simulink library "dcpctrl"  (R2016b)
settings: Solver=ode45  StartTime=0.0  StopTime=10.0  RelTol=1e-3  EnableMultiTasking=on
undefined symbols (not defined in the file): Humusoft, MF644, robot, ts
libraries: simulink x42, sldrtlib x11, dspsigops x2
settings Model: Creator=julianleland  LastModifiedBy=julianleland
settings DataIOCC: LimitDataPoints=on
settings OptimizationCC: LifeSpan=inf
settings DebuggingCC: AllowSymbolicDim=off  SFUnexpectedBacktrackingDiag=warning  SFNoUnconditionalDefaultTransitionDiag=warning  SFExecutionAtInitializationDiag=none
settings GRTTargetCC: TargetLangStandard=C89/C90 (ANSI)  GeneratePreprocessorConditionals=Disable all
settings ConfigComp: CovMetricSettings=dw  CovHtmlReporting=on  CovSaveCumulativeToWorkspaceVar=on  CovSaveSingleToWorkspaceVar=on  CovExternalEMLEnable=off

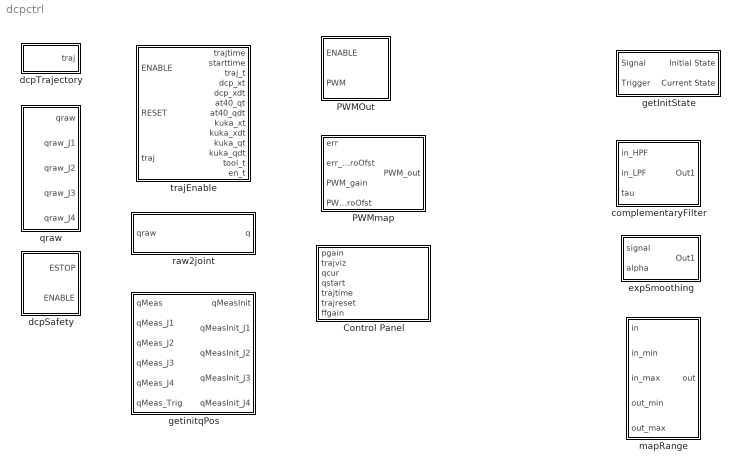
== system dcpctrl ==
  Control Panel : Subsystem
  PWMOut : Subsystem
  PWMmap : Subsystem  mask(PWMmap){}
      mask help:
      | Translates an error signal into a PWM signal, accounting for the dynamics of the AT40GW's PWM interface (deadband, saturation errors).
      |
      | Inputs:
      |  - err: Error signal, unscaled. 4 channels wide.
      |  - err_zeroOfst: Adjusts error "zero" band. A positive number X at this port will cause error values within X of zero to be treated as zero. Default input should be zero.
      |  - PWM_gain: Gain term applied to error signal before conversion to PWM signal. Use this input to scale all PWM signals. Default input should be 1
      |  - PWM_zeroOfst: Adjusts offset of deadband. Positive values will cause deadband limits to increase or decrease. Default input should be zero.
  complementaryFilter : Subsystem
  dcpSafety : Subsystem
  dcpTrajectory : Subsystem
  expSmoothing : Subsystem
  getInitState : Subsystem
  getinitqPos : Subsystem
  "mapRange " : MATLAB Function  TreatAsAtomicUnit=on
  qraw : Subsystem
  raw2joint : Subsystem
  trajEnable : Subsystem

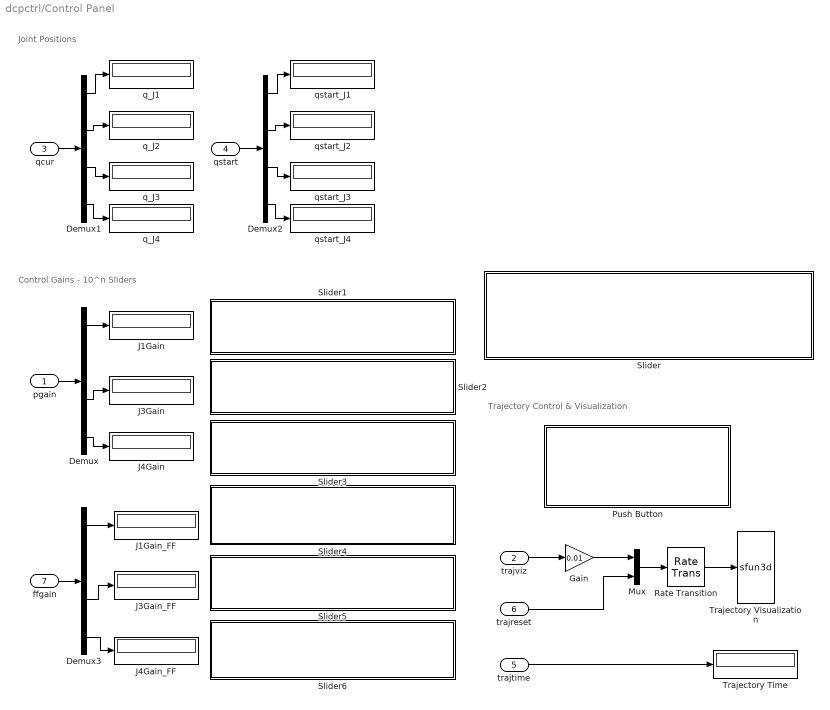
== system dcpctrl/Control Panel ==
  note: Control Gains - 10^n Sliders
  note: Trajectory Control & Visualization
  note: Joint Positions
  pgain : Inport
  trajviz : Inport  Port=2
  qcur : Inport  Port=3
  qstart : Inport  Port=4
  trajtime : Inport  Port=5
  trajreset : Inport  Port=6
  ffgain : Inport  Port=7
  Demux{,1..3} (4 alike) : Demux
  Gain : Gain  Gain=0.01
  J1Gain : Display
  J1Gain_FF : Display
  J3Gain : Display
  J3Gain_FF : Display
  J4Gain : Display
  J4Gain_FF : Display
  Mux : Mux  Inputs=2
  Push Button : Subsystem  DialogController=hmiCreateDDGDialog  IsWebBlock=on  mask(MWDashboardBlock){webBlockId=d14440dc-dcfb-4a22-9820-9883405fda4f, webBlockType=pushbutton, ShowInLibBrwoser=on, ShowInitialText=on, HMISrcModelName=[]}
      mask prompts: webBlockId "WebBlock Id"; webBlockType "WebBlock Type"; HMISrcModelName "Source Model"
      mask Help: helpview([docroot '/mapfiles/simulink.map'], 'hmi_push_button')
      mask Display:
      | model = bdroot(gcb);
      | if strcmp(get_param(model,'BlockDiagramType'), 'library')
      |     image([(matlabroot) '/toolbox/simulink/hmi/icons/PushButton.png']);
      | end
  Rate Transition : RateTransition
  Slider : Subsystem  DialogController=hmiCreateDDGDialog  IsWebBlock=on  mask(MWDashboardBlock){webBlockId=f0c68e46-865a-4d96-89a7-5e1e8ebc446d, webBlockType=slider, ShowInLibBrowser=on, ShowInitialText=on, HMISrcModelName=[]}
      mask prompts: webBlockId "WebBlock Id"; webBlockType "WebBlock Type"; HMISrcModelName "Source Model"
      mask Help: helpview([docroot '/mapfiles/simulink.map'], 'hmi_slider')
      mask Display:
      | if strcmp(get_param(bdroot(gcb),'BlockDiagramType'), 'library')
      |     image([(matlabroot) '/toolbox/simulink/hmi/icons/Slider.png']);
      | end
  Slider1 : Subsystem  DialogController=hmiCreateDDGDialog  IsWebBlock=on  mask(MWDashboardBlock){webBlockId=1b4d9833-0382-4353-be8c-f20f38eb9aab, webBlockType=slider, ShowInLibBrowser=on, ShowInitialText=on, HMISrcModelName=[]}
      mask prompts: webBlockId "WebBlock Id"; webBlockType "WebBlock Type"; HMISrcModelName "Source Model"
      mask Help: helpview([docroot '/mapfiles/simulink.map'], 'hmi_slider')
      mask Display:
      | if strcmp(get_param(bdroot(gcb),'BlockDiagramType'), 'library')
      |     image([(matlabroot) '/toolbox/simulink/hmi/icons/Slider.png']);
      | end
  Slider2 : Subsystem  DialogController=hmiCreateDDGDialog  IsWebBlock=on  mask(MWDashboardBlock){webBlockId=cbf9babb-b489-42eb-b20a-0d2a912eb983, webBlockType=slider, ShowInLibBrowser=on, ShowInitialText=on, HMISrcModelName=[]}
      mask prompts: webBlockId "WebBlock Id"; webBlockType "WebBlock Type"; HMISrcModelName "Source Model"
      mask Help: helpview([docroot '/mapfiles/simulink.map'], 'hmi_slider')
      mask Display:
      | if strcmp(get_param(bdroot(gcb),'BlockDiagramType'), 'library')
      |     image([(matlabroot) '/toolbox/simulink/hmi/icons/Slider.png']);
      | end
  Slider3 : Subsystem  DialogController=hmiCreateDDGDialog  IsWebBlock=on  mask(MWDashboardBlock){webBlockId=af3345d3-46b3-4b00-a2f8-3f6dd7fd4884, webBlockType=slider, ShowInLibBrowser=on, ShowInitialText=on, HMISrcModelName=[]}
      mask prompts: webBlockId "WebBlock Id"; webBlockType "WebBlock Type"; HMISrcModelName "Source Model"
      mask Help: helpview([docroot '/mapfiles/simulink.map'], 'hmi_slider')
      mask Display:
      | if strcmp(get_param(bdroot(gcb),'BlockDiagramType'), 'library')
      |     image([(matlabroot) '/toolbox/simulink/hmi/icons/Slider.png']);
      | end
  Slider4 : Subsystem  DialogController=hmiCreateDDGDialog  IsWebBlock=on  mask(MWDashboardBlock){webBlockId=c89750c1-d32c-4c6a-899a-daca88898995, webBlockType=slider, ShowInLibBrowser=on, ShowInitialText=on, HMISrcModelName=[]}
      mask prompts: webBlockId "WebBlock Id"; webBlockType "WebBlock Type"; HMISrcModelName "Source Model"
      mask Help: helpview([docroot '/mapfiles/simulink.map'], 'hmi_slider')
      mask Display:
      | if strcmp(get_param(bdroot(gcb),'BlockDiagramType'), 'library')
      |     image([(matlabroot) '/toolbox/simulink/hmi/icons/Slider.png']);
      | end
  Slider5 : Subsystem  DialogController=hmiCreateDDGDialog  IsWebBlock=on  mask(MWDashboardBlock){webBlockId=a8dd70f1-7c39-409c-bbaa-299b93baa409, webBlockType=slider, ShowInLibBrowser=on, ShowInitialText=on, HMISrcModelName=[]}
      mask prompts: webBlockId "WebBlock Id"; webBlockType "WebBlock Type"; HMISrcModelName "Source Model"
      mask Help: helpview([docroot '/mapfiles/simulink.map'], 'hmi_slider')
      mask Display:
      | if strcmp(get_param(bdroot(gcb),'BlockDiagramType'), 'library')
      |     image([(matlabroot) '/toolbox/simulink/hmi/icons/Slider.png']);
      | end
  Slider6 : Subsystem  DialogController=hmiCreateDDGDialog  IsWebBlock=on  mask(MWDashboardBlock){webBlockId=99b5f6f1-a2e8-44e0-a565-9b4153c34515, webBlockType=slider, ShowInLibBrowser=on, ShowInitialText=on, HMISrcModelName=[]}
      mask prompts: webBlockId "WebBlock Id"; webBlockType "WebBlock Type"; HMISrcModelName "Source Model"
      mask Help: helpview([docroot '/mapfiles/simulink.map'], 'hmi_slider')
      mask Display:
      | if strcmp(get_param(bdroot(gcb),'BlockDiagramType'), 'library')
      |     image([(matlabroot) '/toolbox/simulink/hmi/icons/Slider.png']);
      | end
  Trajectory Time : Display
  Trajectory Visualization : S-Function  LoadFcn=if exist('sfun3d','file'), sfun3d([],[],[],'LoadBlock'); end  FunctionName=sfun3d  Parameters=ax,T,np,cp,gd,ls,mk  SFunctionDeploymentMode=off  EnableBusSupport=off  mask(3D Graph){np=2, ax=[30 80 -20 20 -10 30], cp=[80 10 20], gd=on, ls=-, mk=., T=0.1}
      mask prompts: np "Number of point (lines)"; ax "[xmin xmax  ymin ymax zmin zmax]"; cp "Camera position (use [0 0 1] for 2D XY view)"; gd "Grid (on|off)"; ls "LineStyle"; mk "Marker"; T "Sampling Time"
      mask help:
      | This block plots the position of several points in the XYZ space. The input contains the coordinates of all the points (x1,y1,z1,x2,y2,z2,...).
      | The number of points (lines), the XYZ ranges, camera position, grid, linestyle, marker and sampling time, can be set as mask parameters.
      settings: CopyFcn=if exist('sfun3d','file'), sfun3d([],[],[],'CopyBlock'); end  DeleteFcn=if exist('sfun3d','file'), sfun3d([],[],[],'DeleteBlock'); end  NameChangeFcn=if exist('sfun3d','file'), sfun3d([],[],[],'NameChange'); end
      mask Help:
      | This block plots the position of several points in the XYZ space. The input contains the coordinates of all the points (x1,y1,z1,x2,y2,z2,...).
      | The number of points (lines), the XYZ ranges, camera position, grid, linestyle, marker and sampling time, can be set as mask parameters.
      mask TypeOptions ls: - | -- | : | -. | none
      mask TypeOptions mk: none | . | + | o | * | x | square | diamond | v | ^ | > | < | pentagram | hexagram
      mask Display: plot([.05 .95 .95 .05 .05],[.45 .45 .95 .95 .45], 0.5+cos(0:0.1:2*pi)*0.3,0.7+sin(0:0.1:2*pi)*0.2)
  q_J{1..4} (4 alike) : Display
  qstart_J{1..4} (4 alike) : Display
  wires:
  trajreset/1 -> Mux/2
  Rate Transition/1 -> Trajectory Visualization/1
  Mux/1 -> Rate Transition/1
  Gain/1 -> Mux/1
  trajviz/1 -> Gain/1
  Demux3/3 -> J3Gain_FF/1
  Demux3/1 -> J1Gain_FF/1
  Demux3/4 -> J4Gain_FF/1
  ffgain/1 -> Demux3/1
  trajtime/1 -> Trajectory Time/1
  Demux2/2 -> qstart_J2/1
  Demux2/3 -> qstart_J3/1
  Demux2/1 -> qstart_J1/1
  Demux2/4 -> qstart_J4/1
  qstart/1 -> Demux2/1
  Demux1/2 -> q_J2/1
  Demux1/3 -> q_J3/1
  Demux1/1 -> q_J1/1
  Demux1/4 -> q_J4/1
  qcur/1 -> Demux1/1
  Demux/3 -> J3Gain/1
  Demux/1 -> J1Gain/1
  Demux/4 -> J4Gain/1
  pgain/1 -> Demux/1

== system dcpctrl/PWMOut ==
  ENABLE : Inport
  "PWM " : Inport  Port=2
  Demux : Demux
  PWM_zero : Constant  Value=robot.Joint(:).PWM_zero
  Switch : Switch  Criteria=u2 ~= 0
  T0Out_PWM : sldrtlib/Frequency Output  SampleTime=-1  MaxMissedTicks=10  ShowMissedTicks=off  YieldWhenWaiting=off  DrvName=Humusoft/MF644  DrvAddress=4294967295  DrvOptions=585  Channels=1  FrequencySource=1  Frequency=500  FrequencyFinalValue=[]  DutySource=2  Duty=0.5  DutyFinalValue=0.5
      settings: AttributesFormatString=Humusoft\nMF644 [auto]
  T1Out_PWM : sldrtlib/Frequency Output  SampleTime=-1  MaxMissedTicks=10  ShowMissedTicks=off  YieldWhenWaiting=off  DrvName=Humusoft/MF644  DrvAddress=4294967295  DrvOptions=585  Channels=2  FrequencySource=1  Frequency=500  FrequencyFinalValue=[]  DutySource=2  Duty=0.5  DutyFinalValue=0.5
      settings: AttributesFormatString=Humusoft\nMF644 [auto]
  T2Out_PWM : sldrtlib/Frequency Output  SampleTime=-1  MaxMissedTicks=10  ShowMissedTicks=off  YieldWhenWaiting=off  DrvName=Humusoft/MF644  DrvAddress=4294967295  DrvOptions=585  Channels=3  FrequencySource=1  Frequency=500  FrequencyFinalValue=[]  DutySource=2  Duty=0.5  DutyFinalValue=0.5
      settings: AttributesFormatString=Humusoft\nMF644 [auto]
  T3Out_PWM : sldrtlib/Frequency Output  SampleTime=-1  MaxMissedTicks=10  ShowMissedTicks=off  YieldWhenWaiting=off  DrvName=Humusoft/MF644  DrvAddress=4294967295  DrvOptions=585  Channels=4  FrequencySource=1  Frequency=500  FrequencyFinalValue=[]  DutySource=2  Duty=0.5  DutyFinalValue=0.5
      settings: AttributesFormatString=Humusoft\nMF644 [auto]
  wires:
  ENABLE/1 -> Switch/2
  PWM_zero/1 -> Switch/3
  "PWM "/1 -> Switch/1
  Switch/1 -> Demux/1
  Demux/1 -> T0Out_PWM/1
  Demux/2 -> T1Out_PWM/1
  Demux/3 -> T2Out_PWM/1
  Demux/4 -> T3Out_PWM/1

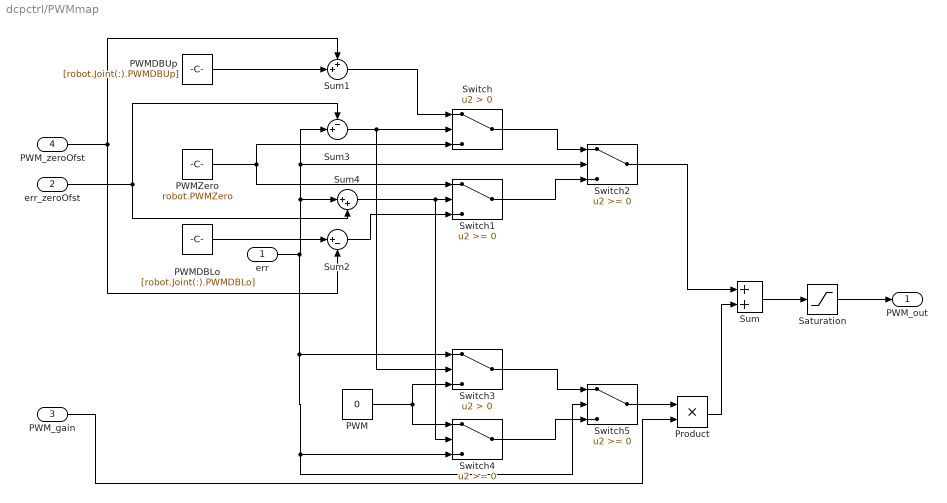
== system dcpctrl/PWMmap ==
  err : Inport
  err_zeroOfst : Inport  Port=2
  "PWM_gain " : Inport  Port=3
  PWM_zeroOfst : Inport  Port=4
  PWM : Constant  Value=0
  PWMDBLo : Constant  Value=[robot.Joint(:).PWMDBLo]
  PWMDBUp : Constant  Value=[robot.Joint(:).PWMDBUp]
  PWMZero : Constant  Value=robot.PWMZero
  Product : Product
  Saturation : Saturate  UpperLimit=[robot.Joint(:).PWMDBMax]  LowerLimit=[robot.Joint(:).PWMDBMin]
  Sum : Sum
  Sum1 : Sum  Inputs=++|
  Sum2 : Sum  Inputs=|+-
  Sum3 : Sum  Inputs=-+|
  Sum4 : Sum  Inputs=|++
  Switch : Switch  Criteria=u2 > Threshold
  Switch{1..2,4..5} (4 alike) : Switch
  Switch3 : Switch  Criteria=u2 > Threshold
  PWM_out : Outport
  wires:
  Switch2/1 -> Sum/1
  Product/1 -> Sum/2
  Sum/1 -> Saturation/1
  Switch5/1 -> Product/1
  PWM/1 -> Switch3/3, Switch4/1
  Switch4/1 -> Switch5/3
  Switch3/1 -> Switch5/1
  Sum1/1 -> Switch/1
  Switch1/1 -> Switch2/3
  Switch/1 -> Switch2/1
  Sum3/1 -> Switch/2, Switch3/2
  Sum4/1 -> Switch1/2, Switch4/2
  err_zeroOfst/1 -> Sum3/1, Sum4/2
  Sum2/1 -> Switch1/3
  PWMDBLo/1 -> Sum2/1
  PWMDBUp/1 -> Sum1/2
  err/1 -> Sum3/2, Switch2/2, Sum4/1, Switch5/2, Switch4/3, Switch3/1
  PWM_zeroOfst/1 -> Sum2/2, Sum1/1
  PWMZero/1 -> Switch/3, Switch1/1
  Saturation/1 -> PWM_out/1
  "PWM_gain "/1 -> Product/2

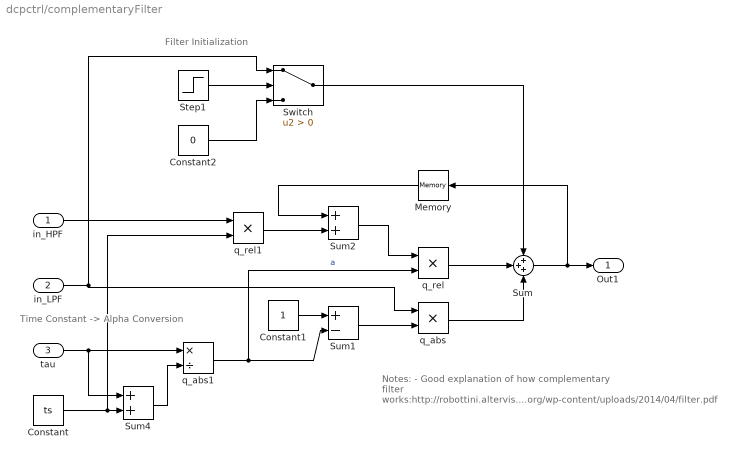
== system dcpctrl/complementaryFilter ==
  note: Notes:
      | - Good explanation of how complementary filter works:http://robottini.altervista.org/wp-content/uploads/2014/04/filter.pdf
  note: Filter Initialization
  note: Time Constant -> Alpha Conversion
  in_HPF : Inport
  "in_LPF " : Inport  Port=2
  tau : Inport  Port=3
  Constant : Constant  Value=ts
  Constant1 : Constant
  Constant2 : Constant  Value=0
  Memory : Memory
  Step1 : Step  Time=ts  Before=1  After=0  SampleTime=0
  Sum : Sum  Inputs=+++
  Sum1 : Sum  Inputs=+-
  Sum2 : Sum
  Sum4 : Sum
  Switch : Switch  Criteria=u2 > Threshold
  q_abs : Product
  q_abs1 : Product  Inputs=*/
  q_rel : Product
  q_rel1 : Product
  Out1 : Outport
  wires:
  Step1/1 -> Switch/2
  Constant2/1 -> Switch/3
  Switch/1 -> Sum/1
  in_HPF/1 -> q_rel1/1
  q_rel1/1 -> Sum2/2
  Constant/1 -> Sum4/2, q_rel1/2
  q_abs1/1 -> Sum1/2, q_rel/2  "a"
  Sum4/1 -> q_abs1/2
  tau/1 -> Sum4/1, q_abs1/1
  Memory/1 -> Sum2/1
  Sum2/1 -> q_rel/1
  q_rel/1 -> Sum/2
  q_abs/1 -> Sum/3
  Constant1/1 -> Sum1/1
  "in_LPF "/1 -> Switch/1, q_abs/1
  Sum1/1 -> q_abs/2
  Sum/1 -> Out1/1, Memory/1

== system dcpctrl/dcpSafety ==
  DIO_ESTOP : sldrtlib/Digital Input  SampleTime=-1  MaxMissedTicks=10  ShowMissedTicks=off  YieldWhenWaiting=off  DrvName=Humusoft/MF644  DrvAddress=4294967295  DrvOptions=585  Channels=1  BitMode=1  DataType=9
      settings: AttributesFormatString=Humusoft\nMF644 [auto]
  DIO_Enable : sldrtlib/Digital Input  SampleTime=-1  MaxMissedTicks=10  ShowMissedTicks=off  YieldWhenWaiting=off  DrvName=Humusoft/MF644  DrvAddress=4294967295  DrvOptions=585  Channels=2  BitMode=1  DataType=9
      settings: AttributesFormatString=Humusoft\nMF644 [auto]
  Logical Operator : Logic  Operator=NOT  AllPortsSameDT=off  OutDataTypeStr=boolean
  ESTOP : Outport
  ENABLE : Outport  Port=2
  wires:
  DIO_ESTOP/1 -> ESTOP/1
  DIO_Enable/1 -> Logical Operator/1
  Logical Operator/1 -> ENABLE/1

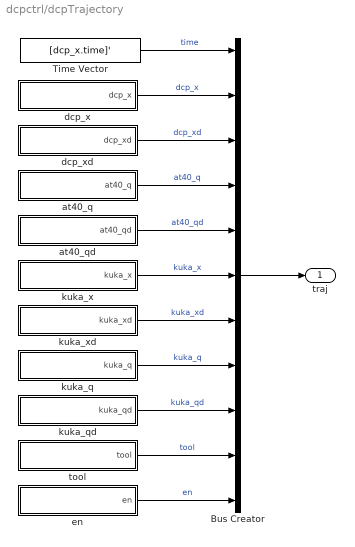
== system dcpctrl/dcpTrajectory ==
  Bus Creator : BusCreator  Inputs=11
  Time Vector : FromWorkspace  VariableName=[dcp_x.time]'  SampleTime=0
  at40_q : Subsystem
  at40_qd : Subsystem
  dcp_x : Subsystem
  dcp_xd : Subsystem
  en : Subsystem
  kuka_q : Subsystem
  kuka_qd : Subsystem
  kuka_x : Subsystem
  kuka_xd : Subsystem
  tool : Subsystem
  traj : Outport
  wires:
  dcp_x/1(dcp_x) -> Bus Creator/2  "dcp_x"
  en/1(en) -> Bus Creator/11  "en"
  tool/1(tool) -> Bus Creator/10  "tool"
  kuka_qd/1(kuka_qd) -> Bus Creator/9  "kuka_qd"
  kuka_q/1(kuka_q) -> Bus Creator/8  "kuka_q"
  kuka_xd/1(kuka_xd) -> Bus Creator/7  "kuka_xd"
  kuka_x/1(kuka_x) -> Bus Creator/6  "kuka_x"
  at40_q/1(at40_q) -> Bus Creator/4  "at40_q"
  Time Vector/1 -> Bus Creator/1  "time"
  dcp_xd/1(dcp_xd) -> Bus Creator/3  "dcp_xd"
  at40_qd/1(at40_qd) -> Bus Creator/5  "at40_qd"
  Bus Creator/1 -> traj/1

== system dcpctrl/expSmoothing ==
  signal : Inport
  alpha : Inport  Port=2
  Constant : Constant
  Memory : Memory
  Product : Product
  Product1 : Product
  Subtract : Sum  Inputs=+-
  Sum : Sum  Inputs=|++
  Out1 : Outport
  wires:
  Subtract/1 -> Product/2
  signal/1 -> Product1/1
  Memory/1 -> Product/1
  alpha/1 -> Subtract/2, Product1/2
  Product1/1 -> Sum/1
  Product/1 -> Sum/2
  Sum/1 -> Out1/1, Memory/1
  Constant/1 -> Subtract/1

== system dcpctrl/getInitState ==
  Signal : Inport
  Trigger : Inport  Port=2
  Delay : Delay  DelayLength=1  InitialCondition=0
  Enabled Subsystem : Subsystem  TreatAsAtomicUnit=on
  Initial State : Outport
  Current State : Outport  Port=2
  wires:
  Delay/1 -> Enabled Subsystem/1(Trigger)
  Trigger/1 -> Enabled Subsystem/Enable, Delay/1
  Enabled Subsystem/2(Cur_State) -> Current State/1
  Enabled Subsystem/1(Init_State) -> Initial State/1
  Signal/1 -> Enabled Subsystem/2(Signal)

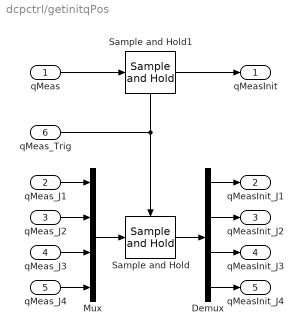
== system dcpctrl/getinitqPos ==
  qMeas : Inport
  qMeas_J1 : Inport  Port=2
  qMeas_J2 : Inport  Port=3
  qMeas_J3 : Inport  Port=4
  qMeas_J4 : Inport  Port=5
  qMeas_Trig : Inport  Port=6
  Demux : Demux
  Mux : Mux
  Sample and Hold : dspsigops/Sample and Hold  trig=Rising edge  initCond=0  latchinput=off
  Sample and Hold1 : dspsigops/Sample and Hold  trig=Rising edge  initCond=0  latchinput=off
  qMeasInit : Outport
  qMeasInit_J1 : Outport  Port=2
  qMeasInit_J2 : Outport  Port=3
  qMeasInit_J3 : Outport  Port=4
  qMeasInit_J4 : Outport  Port=5
  wires:
  qMeas_Trig/1 -> Sample and Hold/Trigger, Sample and Hold1/Trigger
  qMeas_J4/1 -> Mux/4
  qMeas_J3/1 -> Mux/3
  qMeas_J2/1 -> Mux/2
  qMeas_J1/1 -> Mux/1
  Demux/2 -> qMeasInit_J2/1
  Demux/3 -> qMeasInit_J3/1
  Demux/4 -> qMeasInit_J4/1
  Demux/1 -> qMeasInit_J1/1
  Sample and Hold/1 -> Demux/1
  Mux/1 -> Sample and Hold/1
  Sample and Hold1/1 -> qMeasInit/1
  qMeas/1 -> Sample and Hold1/1

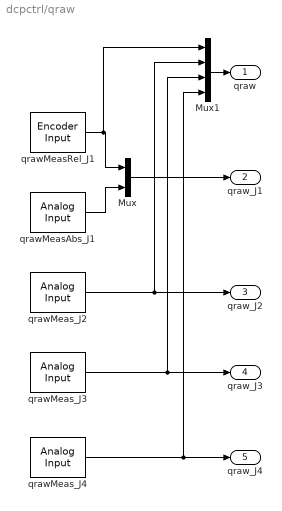
== system dcpctrl/qraw ==
  Mux : Mux  Inputs=2
  Mux1 : Mux
  qrawMeasAbs_J1 : sldrtlib/Analog Input  SampleTime=-1  MaxMissedTicks=10  ShowMissedTicks=off  YieldWhenWaiting=off  DrvName=Humusoft/MF644  DrvAddress=4294967295  DrvOptions=585  Channels=1  RangeMode=1  VoltRange=1  DataType=1
      settings: AttributesFormatString=Humusoft\nMF644 [auto]
  qrawMeasRel_J1 : sldrtlib/Encoder Input  SampleTime=-1  MaxMissedTicks=10  ShowMissedTicks=off  YieldWhenWaiting=off  DrvName=Humusoft/MF644  DrvAddress=4294967295  DrvOptions=585  Channels=1  QuadMode=3  IndexPulse=2  InputFilter=Inf  DataType=1
      settings: AttributesFormatString=Humusoft\nMF644 [auto]
  qrawMeas_J2 : sldrtlib/Analog Input  SampleTime=-1  MaxMissedTicks=10  ShowMissedTicks=off  YieldWhenWaiting=off  DrvName=Humusoft/MF644  DrvAddress=4294967295  DrvOptions=585  Channels=2  RangeMode=1  VoltRange=1  DataType=1
      settings: AttributesFormatString=Humusoft\nMF644 [auto]
  qrawMeas_J3 : sldrtlib/Analog Input  SampleTime=-1  MaxMissedTicks=10  ShowMissedTicks=off  YieldWhenWaiting=off  DrvName=Humusoft/MF644  DrvAddress=4294967295  DrvOptions=585  Channels=3  RangeMode=1  VoltRange=1  DataType=1
      settings: AttributesFormatString=Humusoft\nMF644 [auto]
  qrawMeas_J4 : sldrtlib/Analog Input  SampleTime=-1  MaxMissedTicks=10  ShowMissedTicks=off  YieldWhenWaiting=off  DrvName=Humusoft/MF644  DrvAddress=4294967295  DrvOptions=585  Channels=4  RangeMode=1  VoltRange=1  DataType=1
      settings: AttributesFormatString=Humusoft\nMF644 [auto]
  qraw : Outport
  qraw_J1 : Outport  Port=2
  qraw_J2 : Outport  Port=3
  qraw_J3 : Outport  Port=4
  qraw_J4 : Outport  Port=5
  wires:
  qrawMeas_J4/1 -> Mux1/4, qraw_J4/1
  qrawMeas_J2/1 -> Mux1/2, qraw_J2/1
  qrawMeas_J3/1 -> Mux1/3, qraw_J3/1
  qrawMeasRel_J1/1 -> Mux1/1, Mux/1
  qrawMeasAbs_J1/1 -> Mux/2
  Mux/1 -> qraw_J1/1
  Mux1/1 -> qraw/1

== system dcpctrl/raw2joint ==
  qraw : Inport
  Gain : Gain  Commented=on  Gain=360/robot.Joint(1).PosSensParams.CountsRev
  MATLAB Function : MATLAB Function  TreatAsAtomicUnit=on
  raw2joint_J3 : Subsystem  Commented=on
  raw2joint_J4 : Subsystem  Commented=on
  q : Outport
  wires:
  qraw/1 -> MATLAB Function/1(u)
  MATLAB Function/1(y) -> q/1

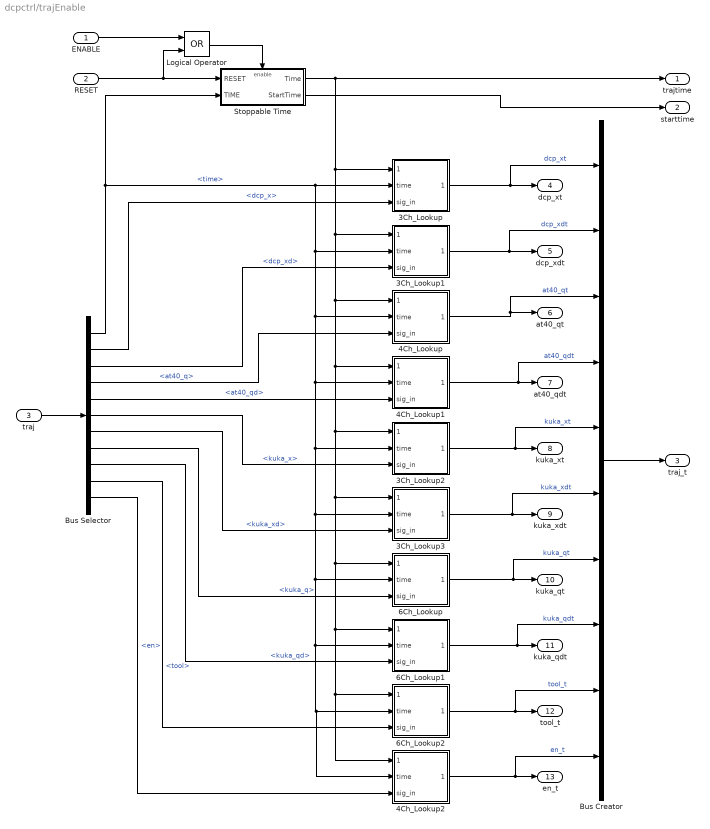
== system dcpctrl/trajEnable ==
  ENABLE : Inport
  RESET : Inport  Port=2
  traj : Inport  Port=3
  3Ch_Lookup : Subsystem
  3Ch_Lookup1 : Subsystem
  3Ch_Lookup2 : Subsystem
  3Ch_Lookup3 : Subsystem
  4Ch_Lookup : Subsystem
  4Ch_Lookup1 : Subsystem
  4Ch_Lookup2 : Subsystem
  6Ch_Lookup : Subsystem
  6Ch_Lookup1 : Subsystem
  6Ch_Lookup2 : Subsystem
  Bus Creator : BusCreator  Inputs=10
  Bus Selector : BusSelector  OutputSignals=time,dcp_x,dcp_xd,at40_q,at40_qd,kuka_x,kuka_xd,kuka_q,kuka_qd,tool,en
  Logical Operator : Logic  Operator=OR  AllPortsSameDT=off  OutDataTypeStr=boolean
  Stoppable Time : Subsystem  TreatAsAtomicUnit=on
  trajtime : Outport
  starttime : Outport  Port=2
  traj_t : Outport  Port=3
  dcp_xt : Outport  Port=4
  dcp_xdt : Outport  Port=5
  at40_qt : Outport  Port=6
  at40_qdt : Outport  Port=7
  kuka_xt : Outport  Port=8
  kuka_xdt : Outport  Port=9
  kuka_qt : Outport  Port=10
  kuka_qdt : Outport  Port=11
  tool_t : Outport  Port=12
  en_t : Outport  Port=13
  wires:
  Stoppable Time/2(StartTime) -> starttime/1
  Bus Creator/1 -> traj_t/1
  4Ch_Lookup2/1(sig_out) -> en_t/1, Bus Creator/10  "en_t"
  6Ch_Lookup1/1(sig_out) -> kuka_qdt/1, Bus Creator/8  "kuka_qdt"
  6Ch_Lookup2/1(sig_out) -> tool_t/1, Bus Creator/9  "tool_t"
  6Ch_Lookup/1(sig_out) -> kuka_qt/1, Bus Creator/7  "kuka_qt"
  3Ch_Lookup3/1(sig_out) -> kuka_xdt/1, Bus Creator/6  "kuka_xdt"
  3Ch_Lookup2/1(sig_out) -> kuka_xt/1, Bus Creator/5  "kuka_xt"
  4Ch_Lookup1/1(sig_out) -> at40_qdt/1, Bus Creator/4  "at40_qdt"
  3Ch_Lookup1/1(sig_out) -> dcp_xdt/1, Bus Creator/2  "dcp_xdt"
  4Ch_Lookup/1(sig_out) -> at40_qt/1, Bus Creator/3  "at40_qt"
  3Ch_Lookup/1(sig_out) -> dcp_xt/1, Bus Creator/1  "dcp_xt"
  Bus Selector/10 -> 6Ch_Lookup2/3(sig_in)  "<tool>"
  Bus Selector/11 -> 4Ch_Lookup2/3(sig_in)  "<en>"
  Bus Selector/9 -> 6Ch_Lookup1/3(sig_in)  "<kuka_qd>"
  Bus Selector/8 -> 6Ch_Lookup/3(sig_in)  "<kuka_q>"
  Bus Selector/7 -> 3Ch_Lookup3/3(sig_in)  "<kuka_xd>"
  Bus Selector/6 -> 3Ch_Lookup2/3(sig_in)  "<kuka_x>"
  Bus Selector/5 -> 4Ch_Lookup1/3(sig_in)  "<at40_qd>"
  Bus Selector/4 -> 4Ch_Lookup/3(sig_in)  "<at40_q>"
  Bus Selector/3 -> 3Ch_Lookup1/3(sig_in)  "<dcp_xd>"
  Bus Selector/2 -> 3Ch_Lookup/3(sig_in)  "<dcp_x>"
  Bus Selector/1 -> 3Ch_Lookup/2(time), 3Ch_Lookup1/2(time), 4Ch_Lookup/2(time), 4Ch_Lookup1/2(time), 6Ch_Lookup/2(time), 4Ch_Lookup2/2(time), 6Ch_Lookup2/2(time), 6Ch_Lookup1/2(time), 3Ch_Lookup3/2(time), 3Ch_Lookup2/2(time), Stoppable Time/2(TIME)  "<time>"
  Logical Operator/1 -> Stoppable Time/Enable
  ENABLE/1 -> Logical Operator/1
  RESET/1 -> Logical Operator/2, Stoppable Time/1(RESET)
  Stoppable Time/1(Time) -> trajtime/1, 3Ch_Lookup1/1(curTime), 4Ch_Lookup/1(curTime), 3Ch_Lookup2/1(curTime), 6Ch_Lookup/1(curTime), 4Ch_Lookup2/1(curTime), 6Ch_Lookup2/1(curTime), 6Ch_Lookup1/1(curTime), 3Ch_Lookup3/1(curTime), 4Ch_Lookup1/1(curTime), 3Ch_Lookup/1(curTime)
  traj/1 -> Bus Selector/1

== system dcpctrl/Control Panel/Push Button ==

== system dcpctrl/Control Panel/Slider ==

== system dcpctrl/Control Panel/Slider1 ==

== system dcpctrl/Control Panel/Slider2 ==

== system dcpctrl/Control Panel/Slider3 ==

== system dcpctrl/Control Panel/Slider4 ==

== system dcpctrl/Control Panel/Slider5 ==

== system dcpctrl/Control Panel/Slider6 ==

== system dcpctrl/dcpTrajectory/at40_q ==
  Mux : Mux
  at40_q1 : FromWorkspace  VariableName=at40_q.data(:,1)'  SampleTime=0
  at40_q2 : FromWorkspace  VariableName=at40_q.data(:,2)'  SampleTime=0
  at40_q3 : FromWorkspace  VariableName=at40_q.data(:,3)'  SampleTime=0
  at40_q4 : FromWorkspace  VariableName=at40_q.data(:,4)'  SampleTime=0
  at40_q : Outport
  wires:
  at40_q4/1 -> Mux/4
  at40_q3/1 -> Mux/3
  at40_q1/1 -> Mux/1
  at40_q2/1 -> Mux/2
  Mux/1 -> at40_q/1  "at40_q"

== system dcpctrl/dcpTrajectory/at40_qd ==
  Mux : Mux
  at40_qd1 : FromWorkspace  VariableName=at40_qd.data(:,1)'  SampleTime=0
  at40_qd2 : FromWorkspace  VariableName=at40_qd.data(:,2)'  SampleTime=0
  at40_qd3 : FromWorkspace  VariableName=at40_qd.data(:,3)'  SampleTime=0
  at40_qd4 : FromWorkspace  VariableName=at40_qd.data(:,4)'  SampleTime=0
  at40_qd : Outport
  wires:
  at40_qd4/1 -> Mux/4
  at40_qd3/1 -> Mux/3
  at40_qd1/1 -> Mux/1
  at40_qd2/1 -> Mux/2
  Mux/1 -> at40_qd/1  "at40_qd"

== system dcpctrl/dcpTrajectory/dcp_x ==
  Mux : Mux  Inputs=3
  dcp_x1 : FromWorkspace  VariableName=dcp_x.data(:,1)'  SampleTime=0
  dcp_x2 : FromWorkspace  VariableName=dcp_x.data(:,2)'  SampleTime=0
  dcp_x3 : FromWorkspace  VariableName=dcp_x.data(:,3)'  SampleTime=0
  dcp_x : Outport
  wires:
  dcp_x3/1 -> Mux/3
  dcp_x1/1 -> Mux/1
  dcp_x2/1 -> Mux/2
  Mux/1 -> dcp_x/1  "dcp_x"

== system dcpctrl/dcpTrajectory/dcp_xd ==
  Mux : Mux  Inputs=3
  dcp_x1 : FromWorkspace  VariableName=dcp_xd.data(:,1)'  SampleTime=0
  dcp_x2 : FromWorkspace  VariableName=dcp_xd.data(:,2)'  SampleTime=0
  dcp_x3 : FromWorkspace  VariableName=dcp_xd.data(:,3)'  SampleTime=0
  dcp_xd : Outport
  wires:
  dcp_x3/1 -> Mux/3
  dcp_x1/1 -> Mux/1
  dcp_x2/1 -> Mux/2
  Mux/1 -> dcp_xd/1  "dcp_xd"

== system dcpctrl/dcpTrajectory/en ==
  Mux : Mux
  en_1 : FromWorkspace  VariableName=en.data(:,1)'  SampleTime=0
  en_2 : FromWorkspace  VariableName=en.data(:,2)'  SampleTime=0
  en_3 : FromWorkspace  VariableName=en.data(:,3)'  SampleTime=0
  en_4 : FromWorkspace  VariableName=en.data(:,4)'  SampleTime=0
  en : Outport
  wires:
  en_4/1 -> Mux/4
  en_3/1 -> Mux/3
  en_1/1 -> Mux/1
  en_2/1 -> Mux/2
  Mux/1 -> en/1  "en"

== system dcpctrl/dcpTrajectory/kuka_q ==
  Mux : Mux  Inputs=6
  kuka_q1 : FromWorkspace  VariableName=kuka_q.data(:,1)'  SampleTime=0
  kuka_q2 : FromWorkspace  VariableName=kuka_q.data(:,2)'  SampleTime=0
  kuka_q3 : FromWorkspace  VariableName=kuka_q.data(:,3)'  SampleTime=0
  kuka_q4 : FromWorkspace  VariableName=kuka_q.data(:,4)'  SampleTime=0
  kuka_q5 : FromWorkspace  VariableName=kuka_q.data(:,5)'  SampleTime=0
  kuka_q6 : FromWorkspace  VariableName=kuka_q.data(:,6)'  SampleTime=0
  kuka_q : Outport
  wires:
  kuka_q6/1 -> Mux/6
  kuka_q5/1 -> Mux/5
  kuka_q4/1 -> Mux/4
  kuka_q3/1 -> Mux/3
  kuka_q1/1 -> Mux/1
  kuka_q2/1 -> Mux/2
  Mux/1 -> kuka_q/1  "kuka_q"

== system dcpctrl/dcpTrajectory/kuka_qd ==
  Mux : Mux  Inputs=6
  kuka_qd1 : FromWorkspace  VariableName=kuka_qd.data(:,1)'  SampleTime=0
  kuka_qd2 : FromWorkspace  VariableName=kuka_qd.data(:,2)'  SampleTime=0
  kuka_qd3 : FromWorkspace  VariableName=kuka_qd.data(:,3)'  SampleTime=0
  kuka_qd4 : FromWorkspace  VariableName=kuka_qd.data(:,4)'  SampleTime=0
  kuka_qd5 : FromWorkspace  VariableName=kuka_qd.data(:,5)'  SampleTime=0
  kuka_qd6 : FromWorkspace  VariableName=kuka_qd.data(:,6)'  SampleTime=0
  kuka_qd : Outport
  wires:
  kuka_qd6/1 -> Mux/6
  kuka_qd5/1 -> Mux/5
  kuka_qd4/1 -> Mux/4
  kuka_qd3/1 -> Mux/3
  kuka_qd1/1 -> Mux/1
  kuka_qd2/1 -> Mux/2
  Mux/1 -> kuka_qd/1  "kuka_qd"

== system dcpctrl/dcpTrajectory/kuka_x ==
  Mux : Mux  Inputs=3
  kuka_x1 : FromWorkspace  VariableName=kuka_x.data(:,1)'  SampleTime=0
  kuka_x2 : FromWorkspace  VariableName=kuka_x.data(:,2)'  SampleTime=0
  kuka_x3 : FromWorkspace  VariableName=kuka_x.data(:,3)'  SampleTime=0
  kuka_x : Outport
  wires:
  kuka_x3/1 -> Mux/3
  kuka_x1/1 -> Mux/1
  kuka_x2/1 -> Mux/2
  Mux/1 -> kuka_x/1  "kuka_x"

== system dcpctrl/dcpTrajectory/kuka_xd ==
  Mux : Mux  Inputs=3
  kuka_xd1 : FromWorkspace  VariableName=kuka_xd.data(:,1)'  SampleTime=0
  kuka_xd2 : FromWorkspace  VariableName=kuka_xd.data(:,2)'  SampleTime=0
  kuka_xd3 : FromWorkspace  VariableName=kuka_xd.data(:,3)'  SampleTime=0
  kuka_xd : Outport
  wires:
  kuka_xd3/1 -> Mux/3
  kuka_xd1/1 -> Mux/1
  kuka_xd2/1 -> Mux/2
  Mux/1 -> kuka_xd/1  "kuka_xd"

== system dcpctrl/dcpTrajectory/tool ==
  Mux : Mux  Inputs=6
  tool_1 : FromWorkspace  VariableName=tool.data(:,1)'  SampleTime=0
  tool_2 : FromWorkspace  VariableName=tool.data(:,2)'  SampleTime=0
  tool_3 : FromWorkspace  VariableName=tool.data(:,3)'  SampleTime=0
  tool_4 : FromWorkspace  VariableName=tool.data(:,4)'  SampleTime=0
  tool_5 : FromWorkspace  VariableName=tool.data(:,5)'  SampleTime=0
  tool_6 : FromWorkspace  VariableName=tool.data(:,6)'  SampleTime=0
  tool : Outport
  wires:
  tool_6/1 -> Mux/6
  tool_5/1 -> Mux/5
  tool_4/1 -> Mux/4
  tool_3/1 -> Mux/3
  tool_1/1 -> Mux/1
  tool_2/1 -> Mux/2
  Mux/1 -> tool/1  "tool"

== system dcpctrl/getInitState/Enabled Subsystem ==
  Trigger : Inport
  Signal : Inport  Port=2
  Enable : EnablePort  StatesWhenEnabling=reset
  Data Type Conversion : DataTypeConversion  OutDataTypeStr=boolean
  IC=ic : Memory  LinearizeAsDelay=on
  Logical Operator : Logic  Operator=NOT  AllPortsSameDT=off  OutDataTypeStr=boolean
  Switch : Switch  Threshold=0.5  SaturateOnIntegerOverflow=on  InputSameDT=on
  Init_State : Outport
  Cur_State : Outport  Port=2
  wires:
  Signal/1 -> Switch/1, Cur_State/1
  Logical Operator/1 -> Data Type Conversion/1
  IC=ic/1 -> Switch/3
  Switch/1 -> Init_State/1, IC=ic/1
  Data Type Conversion/1 -> Switch/2
  Trigger/1 -> Logical Operator/1

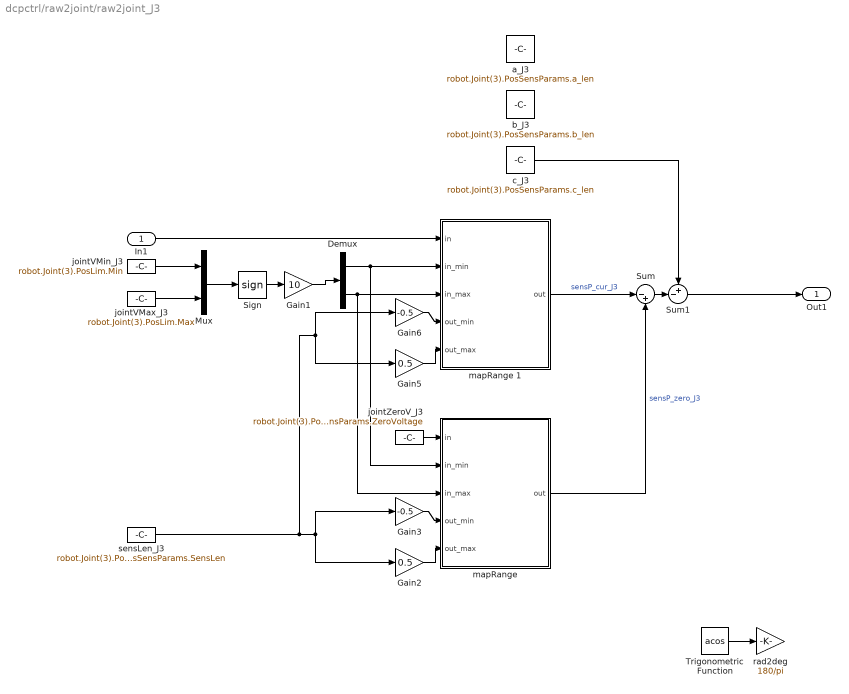
== system dcpctrl/raw2joint/raw2joint_J3 ==
  In1 : Inport
  Demux : Demux  Outputs=2
  Gain1 : Gain  Gain=10
  Gain2 : Gain  Gain=0.5
  Gain3 : Gain  Gain=-0.5
  Gain5 : Gain  Gain=0.5
  Gain6 : Gain  Gain=-0.5
  Mux : Mux  Inputs=2
  Sign : Signum
  Sum : Sum  Inputs=|-+
  Sum1 : Sum  Inputs=+-|
  Trigonometric Function : Trigonometry  Operator=acos  OutputSignalType=real
  a_J3 : Constant  Value=robot.Joint(3).PosSensParams.a_len
  b_J3 : Constant  Value=robot.Joint(3).PosSensParams.b_len
  c_J3 : Constant  Value=robot.Joint(3).PosSensParams.c_len
  jointVMax_J3 : Constant  Value=robot.Joint(3).PosLim.Max
  jointVMin_J3 : Constant  Value=robot.Joint(3).PosLim.Min
  jointZeroV_J3 : Constant  Value=robot.Joint(3).PosSensParams.ZeroVoltage
  "mapRange " : MATLAB Function  TreatAsAtomicUnit=on
  mapRange 1 : MATLAB Function  TreatAsAtomicUnit=on
  rad2deg : Gain  Gain=180/pi
  sensLen_J3 : Constant  Value=robot.Joint(3).PosSensParams.SensLen
  Out1 : Outport
  wires:
  Trigonometric Function/1 -> rad2deg/1
  Mux/1 -> Sign/1
  Sign/1 -> Gain1/1
  Gain2/1 -> "mapRange "/5(out_max)
  Gain3/1 -> "mapRange "/4(out_min)
  Gain1/1 -> Demux/1
  Demux/1 -> "mapRange "/2(in_min), mapRange 1/2(in_min)
  Demux/2 -> "mapRange "/3(in_max), mapRange 1/3(in_max)
  jointZeroV_J3/1 -> "mapRange "/1(in)
  Gain5/1 -> mapRange 1/5(out_max)
  Gain6/1 -> mapRange 1/4(out_min)
  sensLen_J3/1 -> Gain6/1, Gain5/1, Gain3/1, Gain2/1
  jointVMin_J3/1 -> Mux/1
  jointVMax_J3/1 -> Mux/2
  In1/1 -> mapRange 1/1(in)
  mapRange 1/1(out) -> Sum/1  "sensP_cur_J3"
  "mapRange "/1(out) -> Sum/2  "sensP_zero_J3"
  Sum/1 -> Sum1/2
  c_J3/1 -> Sum1/1
  Sum1/1 -> Out1/1

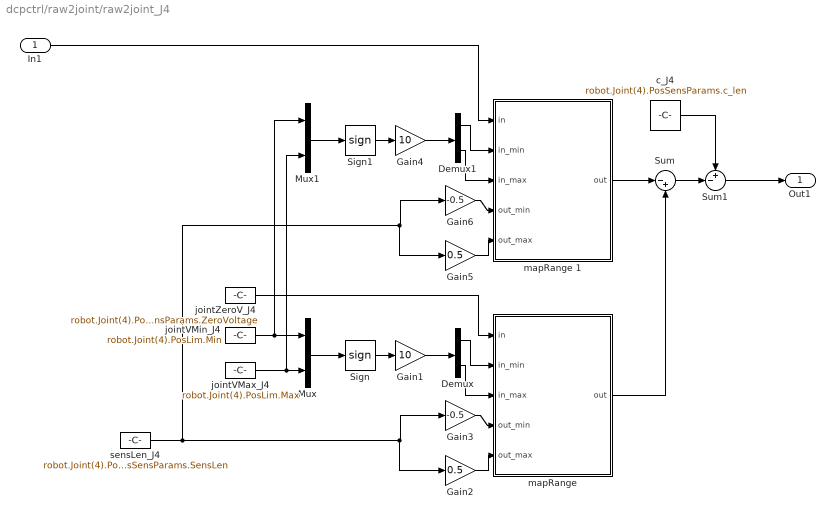
== system dcpctrl/raw2joint/raw2joint_J4 ==
  In1 : Inport
  Demux : Demux  Outputs=2
  Demux1 : Demux  Outputs=2
  Gain1 : Gain  Gain=10
  Gain2 : Gain  Gain=0.5
  Gain3 : Gain  Gain=-0.5
  Gain4 : Gain  Gain=10
  Gain5 : Gain  Gain=0.5
  Gain6 : Gain  Gain=-0.5
  Mux : Mux  Inputs=2
  Mux1 : Mux  Inputs=2
  Sign : Signum
  Sign1 : Signum
  Sum : Sum  Inputs=|-+
  Sum1 : Sum  Inputs=+-|
  c_J4 : Constant  Value=robot.Joint(4).PosSensParams.c_len
  jointVMax_J4 : Constant  Value=robot.Joint(4).PosLim.Max
  jointVMin_J4 : Constant  Value=robot.Joint(4).PosLim.Min
  jointZeroV_J4 : Constant  Value=robot.Joint(4).PosSensParams.ZeroVoltage
  "mapRange " : MATLAB Function  TreatAsAtomicUnit=on
  mapRange 1 : MATLAB Function  TreatAsAtomicUnit=on
  sensLen_J4 : Constant  Value=robot.Joint(4).PosSensParams.SensLen
  Out1 : Outport
  wires:
  Mux/1 -> Sign/1
  Sign/1 -> Gain1/1
  Gain2/1 -> "mapRange "/5(out_max)
  Gain3/1 -> "mapRange "/4(out_min)
  Gain1/1 -> Demux/1
  Demux/1 -> "mapRange "/2(in_min)
  Demux/2 -> "mapRange "/3(in_max)
  jointZeroV_J4/1 -> "mapRange "/1(in)
  Sign1/1 -> Gain4/1
  Gain5/1 -> mapRange 1/5(out_max)
  Gain6/1 -> mapRange 1/4(out_min)
  sensLen_J4/1 -> Gain5/1, Gain6/1, Gain2/1, Gain3/1
  Gain4/1 -> Demux1/1
  jointVMin_J4/1 -> Mux1/1, Mux/1
  jointVMax_J4/1 -> Mux1/2, Mux/2
  Demux1/1 -> mapRange 1/2(in_min)
  Mux1/1 -> Sign1/1
  Demux1/2 -> mapRange 1/3(in_max)
  In1/1 -> mapRange 1/1(in)
  mapRange 1/1(out) -> Sum/1
  "mapRange "/1(out) -> Sum/2
  Sum/1 -> Sum1/2
  c_J4/1 -> Sum1/1
  Sum1/1 -> Out1/1

== system dcpctrl/trajEnable/3Ch_Lookup ==
  curTime : Inport
  time : Inport  Port=2
  sig_in : Inport  Port=3
  Demux : Demux  Outputs=3
  DynLT_Ch1 : simulink/Lookup Tables/Lookup Table Dynamic  LookUpMeth=Interpolation-Use End Values  OutDataTypeStr=fixdt('double')  OutputDataTypeScalingMode=Specify via dialog  OutDataType=fixdt('double')  OutScaling=2^-10  DoSatur=off
  DynLT_Ch2 : simulink/Lookup Tables/Lookup Table Dynamic  LookUpMeth=Interpolation-Use End Values  OutDataTypeStr=fixdt('double')  OutputDataTypeScalingMode=Specify via dialog  OutDataType=fixdt('double')  OutScaling=2^-10  DoSatur=off
  DynLT_Ch3 : simulink/Lookup Tables/Lookup Table Dynamic  LookUpMeth=Interpolation-Use End Values  OutDataTypeStr=fixdt('double')  OutputDataTypeScalingMode=Specify via dialog  OutDataType=fixdt('double')  OutScaling=2^-10  DoSatur=off
  Mux : Mux  Inputs=3
  sig_out : Outport
  wires:
  Mux/1 -> sig_out/1
  sig_in/1 -> Demux/1
  curTime/1 -> DynLT_Ch1/1, DynLT_Ch2/1, DynLT_Ch3/1
  Demux/2 -> DynLT_Ch2/3
  time/1 -> DynLT_Ch1/2, DynLT_Ch2/2, DynLT_Ch3/2
  DynLT_Ch1/1 -> Mux/1
  DynLT_Ch3/1 -> Mux/3
  Demux/1 -> DynLT_Ch1/3
  Demux/3 -> DynLT_Ch3/3
  DynLT_Ch2/1 -> Mux/2

== system dcpctrl/trajEnable/3Ch_Lookup1 ==
  curTime : Inport
  time : Inport  Port=2
  sig_in : Inport  Port=3
  Demux : Demux  Outputs=3
  DynLT_Ch1 : simulink/Lookup Tables/Lookup Table Dynamic  LookUpMeth=Interpolation-Use End Values  OutDataTypeStr=fixdt('double')  OutputDataTypeScalingMode=Specify via dialog  OutDataType=fixdt('double')  OutScaling=2^-10  DoSatur=off
  DynLT_Ch2 : simulink/Lookup Tables/Lookup Table Dynamic  LookUpMeth=Interpolation-Use End Values  OutDataTypeStr=fixdt('double')  OutputDataTypeScalingMode=Specify via dialog  OutDataType=fixdt('double')  OutScaling=2^-10  DoSatur=off
  DynLT_Ch3 : simulink/Lookup Tables/Lookup Table Dynamic  LookUpMeth=Interpolation-Use End Values  OutDataTypeStr=fixdt('double')  OutputDataTypeScalingMode=Specify via dialog  OutDataType=fixdt('double')  OutScaling=2^-10  DoSatur=off
  Mux : Mux  Inputs=3
  sig_out : Outport
  wires:
  Mux/1 -> sig_out/1
  sig_in/1 -> Demux/1
  curTime/1 -> DynLT_Ch1/1, DynLT_Ch2/1, DynLT_Ch3/1
  Demux/2 -> DynLT_Ch2/3
  time/1 -> DynLT_Ch1/2, DynLT_Ch2/2, DynLT_Ch3/2
  DynLT_Ch1/1 -> Mux/1
  DynLT_Ch3/1 -> Mux/3
  Demux/1 -> DynLT_Ch1/3
  Demux/3 -> DynLT_Ch3/3
  DynLT_Ch2/1 -> Mux/2

== system dcpctrl/trajEnable/3Ch_Lookup2 ==
  curTime : Inport
  time : Inport  Port=2
  sig_in : Inport  Port=3
  Demux : Demux  Outputs=3
  DynLT_Ch1 : simulink/Lookup Tables/Lookup Table Dynamic  LookUpMeth=Interpolation-Use End Values  OutDataTypeStr=fixdt('double')  OutputDataTypeScalingMode=Specify via dialog  OutDataType=fixdt('double')  OutScaling=2^-10  DoSatur=off
  DynLT_Ch2 : simulink/Lookup Tables/Lookup Table Dynamic  LookUpMeth=Interpolation-Use End Values  OutDataTypeStr=fixdt('double')  OutputDataTypeScalingMode=Specify via dialog  OutDataType=fixdt('double')  OutScaling=2^-10  DoSatur=off
  DynLT_Ch3 : simulink/Lookup Tables/Lookup Table Dynamic  LookUpMeth=Interpolation-Use End Values  OutDataTypeStr=fixdt('double')  OutputDataTypeScalingMode=Specify via dialog  OutDataType=fixdt('double')  OutScaling=2^-10  DoSatur=off
  Mux : Mux  Inputs=3
  sig_out : Outport
  wires:
  Mux/1 -> sig_out/1
  sig_in/1 -> Demux/1
  curTime/1 -> DynLT_Ch1/1, DynLT_Ch2/1, DynLT_Ch3/1
  Demux/2 -> DynLT_Ch2/3
  time/1 -> DynLT_Ch1/2, DynLT_Ch2/2, DynLT_Ch3/2
  DynLT_Ch1/1 -> Mux/1
  DynLT_Ch3/1 -> Mux/3
  Demux/1 -> DynLT_Ch1/3
  Demux/3 -> DynLT_Ch3/3
  DynLT_Ch2/1 -> Mux/2

== system dcpctrl/trajEnable/3Ch_Lookup3 ==
  curTime : Inport
  time : Inport  Port=2
  sig_in : Inport  Port=3
  Demux : Demux  Outputs=3
  DynLT_Ch1 : simulink/Lookup Tables/Lookup Table Dynamic  LookUpMeth=Interpolation-Use End Values  OutDataTypeStr=fixdt('double')  OutputDataTypeScalingMode=Specify via dialog  OutDataType=fixdt('double')  OutScaling=2^-10  DoSatur=off
  DynLT_Ch2 : simulink/Lookup Tables/Lookup Table Dynamic  LookUpMeth=Interpolation-Use End Values  OutDataTypeStr=fixdt('double')  OutputDataTypeScalingMode=Specify via dialog  OutDataType=fixdt('double')  OutScaling=2^-10  DoSatur=off
  DynLT_Ch3 : simulink/Lookup Tables/Lookup Table Dynamic  LookUpMeth=Interpolation-Use End Values  OutDataTypeStr=fixdt('double')  OutputDataTypeScalingMode=Specify via dialog  OutDataType=fixdt('double')  OutScaling=2^-10  DoSatur=off
  Mux : Mux  Inputs=3
  sig_out : Outport
  wires:
  Mux/1 -> sig_out/1
  sig_in/1 -> Demux/1
  curTime/1 -> DynLT_Ch1/1, DynLT_Ch2/1, DynLT_Ch3/1
  Demux/2 -> DynLT_Ch2/3
  time/1 -> DynLT_Ch1/2, DynLT_Ch2/2, DynLT_Ch3/2
  DynLT_Ch1/1 -> Mux/1
  DynLT_Ch3/1 -> Mux/3
  Demux/1 -> DynLT_Ch1/3
  Demux/3 -> DynLT_Ch3/3
  DynLT_Ch2/1 -> Mux/2

== system dcpctrl/trajEnable/4Ch_Lookup ==
  curTime : Inport
  time : Inport  Port=2
  sig_in : Inport  Port=3
  Demux : Demux
  DynLT_Ch{1..4} (4 alike) : simulink/Lookup Tables/Lookup Table Dynamic  LookUpMeth=Interpolation-Use End Values  OutDataTypeStr=fixdt('double')  OutputDataTypeScalingMode=Specify via dialog  OutDataType=fixdt('double')  OutScaling=2^-10  DoSatur=off
  Mux : Mux
  sig_out : Outport
  wires:
  DynLT_Ch4/1 -> Mux/4
  DynLT_Ch3/1 -> Mux/3
  Demux/4 -> DynLT_Ch4/3
  Mux/1 -> sig_out/1
  sig_in/1 -> Demux/1
  curTime/1 -> DynLT_Ch1/1, DynLT_Ch2/1, DynLT_Ch3/1, DynLT_Ch4/1
  Demux/2 -> DynLT_Ch2/3
  time/1 -> DynLT_Ch1/2, DynLT_Ch2/2, DynLT_Ch3/2, DynLT_Ch4/2
  DynLT_Ch1/1 -> Mux/1
  Demux/1 -> DynLT_Ch1/3
  Demux/3 -> DynLT_Ch3/3
  DynLT_Ch2/1 -> Mux/2

== system dcpctrl/trajEnable/4Ch_Lookup1 ==
  curTime : Inport
  time : Inport  Port=2
  sig_in : Inport  Port=3
  Demux : Demux
  DynLT_Ch{1..4} (4 alike) : simulink/Lookup Tables/Lookup Table Dynamic  LookUpMeth=Interpolation-Use End Values  OutDataTypeStr=fixdt('double')  OutputDataTypeScalingMode=Specify via dialog  OutDataType=fixdt('double')  OutScaling=2^-10  DoSatur=off
  Mux : Mux
  sig_out : Outport
  wires:
  DynLT_Ch4/1 -> Mux/4
  DynLT_Ch3/1 -> Mux/3
  Demux/4 -> DynLT_Ch4/3
  Mux/1 -> sig_out/1
  sig_in/1 -> Demux/1
  curTime/1 -> DynLT_Ch1/1, DynLT_Ch2/1, DynLT_Ch3/1, DynLT_Ch4/1
  Demux/2 -> DynLT_Ch2/3
  time/1 -> DynLT_Ch1/2, DynLT_Ch2/2, DynLT_Ch3/2, DynLT_Ch4/2
  DynLT_Ch1/1 -> Mux/1
  Demux/1 -> DynLT_Ch1/3
  Demux/3 -> DynLT_Ch3/3
  DynLT_Ch2/1 -> Mux/2

== system dcpctrl/trajEnable/4Ch_Lookup2 ==
  curTime : Inport
  time : Inport  Port=2
  sig_in : Inport  Port=3
  Demux : Demux
  DynLT_Ch{1..4} (4 alike) : simulink/Lookup Tables/Lookup Table Dynamic  LookUpMeth=Interpolation-Use End Values  OutDataTypeStr=fixdt('double')  OutputDataTypeScalingMode=Specify via dialog  OutDataType=fixdt('double')  OutScaling=2^-10  DoSatur=off
  Mux : Mux
  sig_out : Outport
  wires:
  DynLT_Ch4/1 -> Mux/4
  DynLT_Ch3/1 -> Mux/3
  Demux/4 -> DynLT_Ch4/3
  Mux/1 -> sig_out/1
  sig_in/1 -> Demux/1
  curTime/1 -> DynLT_Ch1/1, DynLT_Ch2/1, DynLT_Ch3/1, DynLT_Ch4/1
  Demux/2 -> DynLT_Ch2/3
  time/1 -> DynLT_Ch1/2, DynLT_Ch2/2, DynLT_Ch3/2, DynLT_Ch4/2
  DynLT_Ch1/1 -> Mux/1
  Demux/1 -> DynLT_Ch1/3
  Demux/3 -> DynLT_Ch3/3
  DynLT_Ch2/1 -> Mux/2

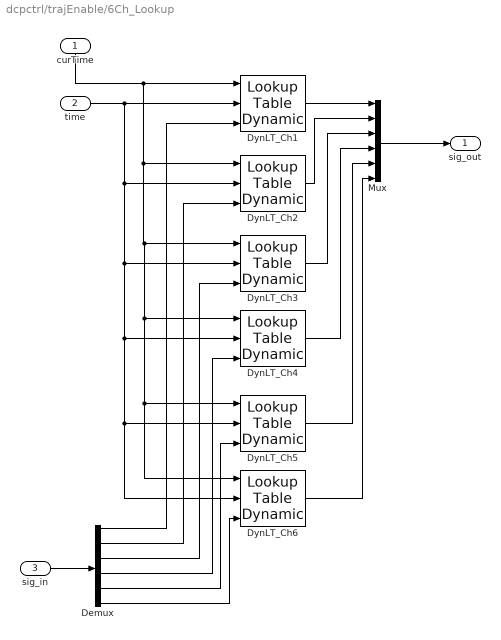
== system dcpctrl/trajEnable/6Ch_Lookup ==
  curTime : Inport
  time : Inport  Port=2
  sig_in : Inport  Port=3
  Demux : Demux  Outputs=6
  DynLT_Ch{1..6} (6 alike) : simulink/Lookup Tables/Lookup Table Dynamic  LookUpMeth=Interpolation-Use End Values  OutDataTypeStr=fixdt('double')  OutputDataTypeScalingMode=Specify via dialog  OutDataType=fixdt('double')  OutScaling=2^-10  DoSatur=off
  Mux : Mux  Inputs=6
  sig_out : Outport
  wires:
  Demux/6 -> DynLT_Ch6/3
  Demux/5 -> DynLT_Ch5/3
  DynLT_Ch6/1 -> Mux/6
  DynLT_Ch5/1 -> Mux/5
  DynLT_Ch4/1 -> Mux/4
  DynLT_Ch3/1 -> Mux/3
  Demux/4 -> DynLT_Ch4/3
  Mux/1 -> sig_out/1
  sig_in/1 -> Demux/1
  curTime/1 -> DynLT_Ch1/1, DynLT_Ch2/1, DynLT_Ch3/1, DynLT_Ch4/1, DynLT_Ch6/1, DynLT_Ch5/1
  Demux/2 -> DynLT_Ch2/3
  time/1 -> DynLT_Ch1/2, DynLT_Ch2/2, DynLT_Ch3/2, DynLT_Ch4/2, DynLT_Ch6/2, DynLT_Ch5/2
  DynLT_Ch1/1 -> Mux/1
  Demux/1 -> DynLT_Ch1/3
  Demux/3 -> DynLT_Ch3/3
  DynLT_Ch2/1 -> Mux/2

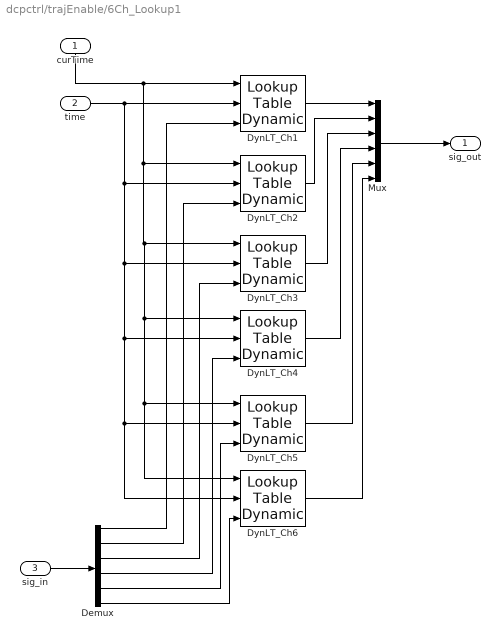
== system dcpctrl/trajEnable/6Ch_Lookup1 ==
  curTime : Inport
  time : Inport  Port=2
  sig_in : Inport  Port=3
  Demux : Demux  Outputs=6
  DynLT_Ch{1..6} (6 alike) : simulink/Lookup Tables/Lookup Table Dynamic  LookUpMeth=Interpolation-Use End Values  OutDataTypeStr=fixdt('double')  OutputDataTypeScalingMode=Specify via dialog  OutDataType=fixdt('double')  OutScaling=2^-10  DoSatur=off
  Mux : Mux  Inputs=6
  sig_out : Outport
  wires:
  Demux/6 -> DynLT_Ch6/3
  Demux/5 -> DynLT_Ch5/3
  DynLT_Ch6/1 -> Mux/6
  DynLT_Ch5/1 -> Mux/5
  DynLT_Ch4/1 -> Mux/4
  DynLT_Ch3/1 -> Mux/3
  Demux/4 -> DynLT_Ch4/3
  Mux/1 -> sig_out/1
  sig_in/1 -> Demux/1
  curTime/1 -> DynLT_Ch1/1, DynLT_Ch2/1, DynLT_Ch3/1, DynLT_Ch4/1, DynLT_Ch6/1, DynLT_Ch5/1
  Demux/2 -> DynLT_Ch2/3
  time/1 -> DynLT_Ch1/2, DynLT_Ch2/2, DynLT_Ch3/2, DynLT_Ch4/2, DynLT_Ch6/2, DynLT_Ch5/2
  DynLT_Ch1/1 -> Mux/1
  Demux/1 -> DynLT_Ch1/3
  Demux/3 -> DynLT_Ch3/3
  DynLT_Ch2/1 -> Mux/2

== system dcpctrl/trajEnable/6Ch_Lookup2 ==
  curTime : Inport
  time : Inport  Port=2
  sig_in : Inport  Port=3
  Demux : Demux  Outputs=6
  DynLT_Ch{1..6} (6 alike) : simulink/Lookup Tables/Lookup Table Dynamic  LookUpMeth=Interpolation-Use End Values  OutDataTypeStr=fixdt('double')  OutputDataTypeScalingMode=Specify via dialog  OutDataType=fixdt('double')  OutScaling=2^-10  DoSatur=off
  Mux : Mux  Inputs=6
  sig_out : Outport
  wires:
  Demux/6 -> DynLT_Ch6/3
  Demux/5 -> DynLT_Ch5/3
  DynLT_Ch6/1 -> Mux/6
  DynLT_Ch5/1 -> Mux/5
  DynLT_Ch4/1 -> Mux/4
  DynLT_Ch3/1 -> Mux/3
  Demux/4 -> DynLT_Ch4/3
  Mux/1 -> sig_out/1
  sig_in/1 -> Demux/1
  curTime/1 -> DynLT_Ch1/1, DynLT_Ch2/1, DynLT_Ch3/1, DynLT_Ch4/1, DynLT_Ch6/1, DynLT_Ch5/1
  Demux/2 -> DynLT_Ch2/3
  time/1 -> DynLT_Ch1/2, DynLT_Ch2/2, DynLT_Ch3/2, DynLT_Ch4/2, DynLT_Ch6/2, DynLT_Ch5/2
  DynLT_Ch1/1 -> Mux/1
  Demux/1 -> DynLT_Ch1/3
  Demux/3 -> DynLT_Ch3/3
  DynLT_Ch2/1 -> Mux/2

== system dcpctrl/trajEnable/Stoppable Time ==
  RESET : Inport
  TIME : Inport  Port=2
  Enable : EnablePort
  Constant : Constant
  Integrator : Integrator  ExternalReset=level hold
  MinMax : MinMax  Function=max
  Sum : Sum  Inputs=|++
  "Trajectory Time " : Gain  Gain=0.1632124352331606
  Time : Outport
  StartTime : Outport  Port=2
  wires:
  MinMax/1 -> "Trajectory Time "/1
  TIME/1 -> MinMax/1
  "Trajectory Time "/1 -> Sum/2, StartTime/1
  Integrator/1 -> Sum/1
  Sum/1 -> Time/1
  RESET/1 -> Integrator/2
  Constant/1 -> Integrator/1

== matlab function dcpctrl/raw2joint/MATLAB Function ==
  data: u input; y output; robot parameter
function y = fcn(u, robot)
%#codegen

y_temp = raw2joint_at40gw(robot,u');
y = y_temp';

== matlab function dcpctrl/raw2joint/raw2joint_J3/mapRange  ==
  data: in input; out output; in_min input; in_max input; out_min input; out_max input
function out = mapRange(in, in_min, in_max, out_min, out_max )
%MAPRANGE Map value from one range to a second range.

% [ out_value ] = mapRange(x, in_min, in_max, out_min, out_max )
%   Julian Leland, MIT Media Lab, 2016-06-07
%   Exact knockoff of Arduino map function - see here for details: 
%   https://www.arduino.cc/en/Reference/Map
%   INPUTS:
%   x - input value to be mapped. May be a vector.
%   in_min - minumum value in range that is being mapped from
%   in_max - maximum value in range that is being mapped from
%   out_min - minimum value in range that is being mapped to
%   out_max - maximum value in range that is being mapped to
%
%   Example usage:
%   foo = [100;5;3]
%   bar = mapRange(foo,0,100,500,1000)
%   bar = [1000;525;515]

out = ((in-in_min).*(out_max-out_min))./(in_max-in_min)+out_min;

end

== matlab function dcpctrl/raw2joint/raw2joint_J3/mapRange 1 ==
  data: in input; out output; in_min input; in_max input; out_min input; out_max input
function out = mapRange(in, in_min, in_max, out_min, out_max )
%MAPRANGE Map value from one range to a second range.

% [ out_value ] = mapRange(x, in_min, in_max, out_min, out_max )
%   Julian Leland, MIT Media Lab, 2016-06-07
%   Exact knockoff of Arduino map function - see here for details: 
%   https://www.arduino.cc/en/Reference/Map
%   INPUTS:
%   x - input value to be mapped. May be a vector.
%   in_min - minumum value in range that is being mapped from
%   in_max - maximum value in range that is being mapped from
%   out_min - minimum value in range that is being mapped to
%   out_max - maximum value in range that is being mapped to
%
%   Example usage:
%   foo = [100;5;3]
%   bar = mapRange(foo,0,100,500,1000)
%   bar = [1000;525;515]

out = ((in-in_min).*(out_max-out_min))./(in_max-in_min)+out_min;

end

== matlab function dcpctrl/mapRange  ==
  data: in input; out output; in_min input; in_max input; out_min input; out_max input
function out = mapRange(in, in_min, in_max, out_min, out_max )
%MAPRANGE Map value from one range to a second range.

% [ out_value ] = mapRange(x, in_min, in_max, out_min, out_max )
%   Julian Leland, MIT Media Lab, 2016-06-07
%   Exact knockoff of Arduino map function - see here for details: 
%   https://www.arduino.cc/en/Reference/Map
%   INPUTS:
%   x - input value to be mapped. May be a vector.
%   in_min - minumum value in range that is being mapped from
%   in_max - maximum value in range that is being mapped from
%   out_min - minimum value in range that is being mapped to
%   out_max - maximum value in range that is being mapped to
%
%   Example usage:
%   foo = [100;5;3]
%   bar = mapRange(foo,0,100,500,1000)
%   bar = [1000;525;515]

out = ((in-in_min).*(out_max-out_min))./(in_max-in_min)+out_min;

end

== matlab function dcpctrl/raw2joint/raw2joint_J4/mapRange  ==
  data: in input; out output; in_min input; in_max input; out_min input; out_max input
function out = mapRange(in, in_min, in_max, out_min, out_max )
%MAPRANGE Map value from one range to a second range.

% [ out_value ] = mapRange(x, in_min, in_max, out_min, out_max )
%   Julian Leland, MIT Media Lab, 2016-06-07
%   Exact knockoff of Arduino map function - see here for details: 
%   https://www.arduino.cc/en/Reference/Map
%   INPUTS:
%   x - input value to be mapped. May be a vector.
%   in_min - minumum value in range that is being mapped from
%   in_max - maximum value in range that is being mapped from
%   out_min - minimum value in range that is being mapped to
%   out_max - maximum value in range that is being mapped to
%
%   Example usage:
%   foo = [100;5;3]
%   bar = mapRange(foo,0,100,500,1000)
%   bar = [1000;525;515]

out = ((in-in_min).*(out_max-out_min))./(in_max-in_min)+out_min;

end

== matlab function dcpctrl/raw2joint/raw2joint_J4/mapRange 1 ==
  data: in input; out output; in_min input; in_max input; out_min input; out_max input
function out = mapRange(in, in_min, in_max, out_min, out_max )
%MAPRANGE Map value from one range to a second range.

% [ out_value ] = mapRange(x, in_min, in_max, out_min, out_max )
%   Julian Leland, MIT Media Lab, 2016-06-07
%   Exact knockoff of Arduino map function - see here for details: 
%   https://www.arduino.cc/en/Reference/Map
%   INPUTS:
%   x - input value to be mapped. May be a vector.
%   in_min - minumum value in range that is being mapped from
%   in_max - maximum value in range that is being mapped from
%   out_min - minimum value in range that is being mapped to
%   out_max - maximum value in range that is being mapped to
%
%   Example usage:
%   foo = [100;5;3]
%   bar = mapRange(foo,0,100,500,1000)
%   bar = [1000;525;515]

out = ((in-in_min).*(out_max-out_min))./(in_max-in_min)+out_min;

end
